simulink model "model_quad_linear_mpc"  (R2021b)
settings: Solver=FixedStepAuto  StartTime=0.0  StopTime=10  FixedStep=.01  RelTol=1e-3
values from neighbouring files (symbols this model uses):
  A = reshape([mt1,mt2,mt3,mt4,mt5,mt6,mt7,mt8],12,12)    [Jacob.m]    (also in Lineared_SS_model.m = reshape([-1.097500e-06;0.000000e+00;0.000000e+00;-4.432200e-; find_optimal_lqr.m = reshape([-1.097500e-06;0.000000e+00;0.000000e+00;-4.432200e-; start_drone.m = zeros(12))
  B = reshape([mt9,mt10],12,4)    [Jacob.m]    (also in Lineared_SS_model.m = reshape([0.000000e+00;0.000000e+00;0.000000e+00;0.000000e+00; find_optimal_lqr.m = reshape([0.000000e+00;0.000000e+00;0.000000e+00;0.000000e+00; nlStateFcn.m = [0 0 0]; start_drone.m = zeros(12,4))
libraries: mpclib x1
settings Model: Creator=Elena  LastModifiedBy=Elena

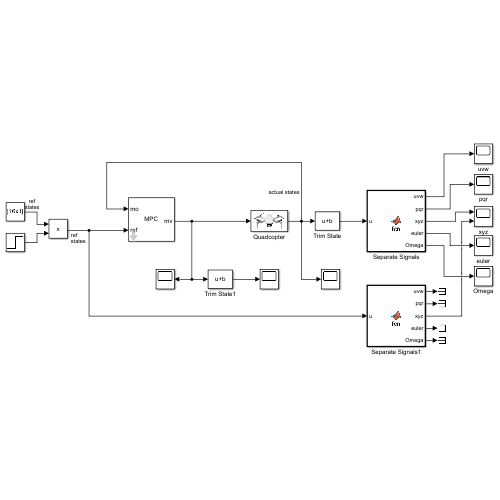
[thumbnail: Simulink's stored preview of the top-level diagram]
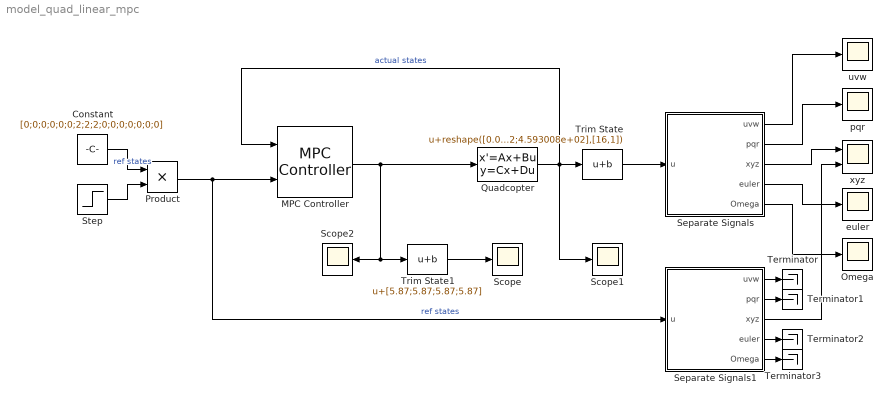
== system model_quad_linear_mpc ==
  Constant : Constant  Value=[0;0;0;0;0;0;2;2;2;0;0;0;0;0;0;0]
  MPC Controller : mpclib/MPC Controller  SCDEnableBlockLinearizationSpecification=on  mpcobj=mpc_l  is_multiple=0  enable_value=0  return_u0=off  updateMPCinCallerWorkspace=on  md_inport=off  mv_inport=off  uref_inport=off  return_cost=off  return_mvseq=off  return_qpstatus=off  return_xseq=off  return_state=off  return_ovseq=off  state_inport=off  umin_inport=off  umax_inport=off  ymin_inport=off  ymax_inport=off  cc_inport=off  ywt_inport=off  uwt_inport=off  duwt_inport=off  rhoeps_inport=off  pm_inport=off  MaximumP=10  HorizonChoice=FixedHorizon  n_ts=0.1  n_p=20  n_mv=4  n_md=0  n_ud=0  n_mo=16  n_uo=0  BlockDataType=double  SampleTimeInherited=off  switch_inport=off
  Omega : Scope
  Product : Product
  Quadcopter : StateSpace  A=A  B=B  C=eye(16)  D=zeros(16,4)  InitialCondition=0
      mask Display: image('drone_model.png'); % Use "Edit Image" on toolstrip to change.
  Scope : Scope
  Scope1 : Scope
  Scope2 : Scope
  Separate Signals : MATLAB Function  TreatAsAtomicUnit=on
  Separate Signals1 : MATLAB Function  TreatAsAtomicUnit=on
  Step : Step  SampleTime=0
  Terminator{,1..3} (4 alike) : Terminator
  Trim State : Bias  Bias=reshape([0.000000e+00;0.000000e+00;0.000000e+00;0.000000e+00;0.000000e+00;0.000000e+00;0.000000e+00;0.000000e+00;0.000000e+00;0.000000e+00;0.000000e+00;0.000000e+00;0;4.593008e+02;4.593008e+02;4.593008e+02],[16,1])
  Trim State1 : Bias  Bias=[5.87;5.87;5.87;5.87]
  euler : Scope
  pqr : Scope
  uvw : Scope
  xyz : Scope  NumInputPorts=2
  wires:
  Step/1 -> Product/2
  Quadcopter/1 -> MPC Controller/1, Trim State/1, Scope1/1  "actual states"
  Separate Signals/3(xyz) -> xyz/1
  Separate Signals/2(pqr) -> pqr/1
  Separate Signals/1(uvw) -> uvw/1
  Separate Signals/4(euler) -> euler/1
  Separate Signals/5(Omega) -> Omega/1
  Trim State/1 -> Separate Signals/1(u)
  Separate Signals1/3(xyz) -> xyz/2
  Separate Signals1/1(uvw) -> Terminator/1
  Separate Signals1/2(pqr) -> Terminator1/1
  Separate Signals1/4(euler) -> Terminator2/1
  Separate Signals1/5(Omega) -> Terminator3/1
  Product/1 -> Separate Signals1/1(u), MPC Controller/2  "ref states"
  Constant/1 -> Product/1  "ref states"
  MPC Controller/1 -> Scope2/1, Trim State1/1, Quadcopter/1
  Trim State1/1 -> Scope/1

== matlab function model_quad_linear_mpc/Separate Signals1 ==
  data: u input; uvw output; pqr output; xyz output; euler output; Omega output
function [uvw,pqr,xyz,euler,Omega] = fcn(u)

uvw=u(1:3);
pqr=u((1:3)+3);
xyz=u((1:3)+6);
euler=u((1:3)+9);
Omega=u((1:4)+12);

== matlab function model_quad_linear_mpc/Separate Signals ==
  data: u input; uvw output; pqr output; xyz output; euler output; Omega output
function [uvw,pqr,xyz,euler,Omega] = fcn(u)

uvw=u(1:3);
pqr=u((1:3)+3);
xyz=u((1:3)+6);
euler=u((1:3)+9);
Omega=u((1:4)+12);
